simulink model "Hardmon"  (R2025b)
settings: Solver=ode8  StartTime=0.0  StopTime=10  FixedStep=0.0001  RelTol=1e-3
undefined symbols (not defined in the file or in its folder): BMS_Contactor_Command
settings Model: DataDictionary=rev3_data.sldd  Creator=heyka  LastModifiedBy=ryanz
settings DataIOCC: ExternalInput=test_temp.getElement('Temp 1'),test_temp.getElement('Temp 2')  LoadExternalInput=on
settings OptimizationCC: DefaultParameterBehavior=Inlined  EnhancedBackFolding=on  PassReuseOutputArgsThreshold=0.0  ZeroExternalMemoryAtStartup=off  ZeroInternalMemoryAtStartup=off  OptimizeBlockOrder=speed  DifferentSizesBufferReuse=on  OptimizationCustomize=off
settings DebuggingCC: SolverPrmCheckMsg=warning  ParameterTunabilityLossMsg=error  StateNameClashWarn=warning
settings HardwareCC: ProdBitPerInt=16.0  ProdBitPerPointer=16.0  ProdBitPerSizeT=16.0  ProdBitPerPtrDiffT=16.0  ProdLargestAtomicFloat=None  ProdWordSize=16.0  ProdHWDeviceType=STMicroelectronics->ST10/Super10
settings SFSimCC: MATLABDynamicMemAlloc=off  SimTargetLang=C++  SimDLTargetLibrary=mkl-dnn
settings RTWCC: GenCodeOnly=on  Toolchain=MinGW64 | gmake (64-bit Windows)  BuildConfiguration=Faster Runs  TargetLang=C++  GPUComputeCapability=3.5
settings CodeAppCC: ForceParamTrailComments=on  OperatorAnnotations=on  StateflowObjectComments=on
settings GRTTargetCC: TargetLangStandard=C++11 (ISO)  CodeInterfacePackaging=C++ class  SubcomponentCodeInterfacePackaging=C++ class

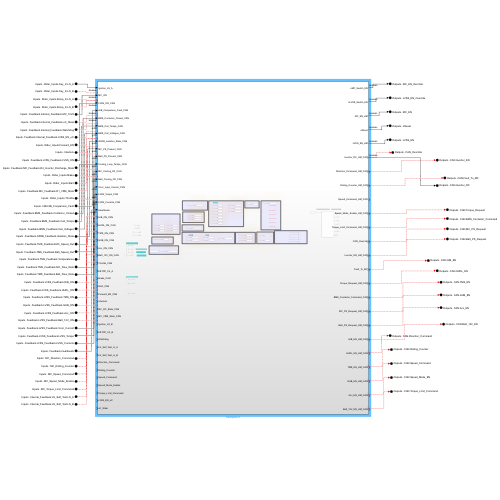
[thumbnail: Simulink's stored preview of the top-level diagram]
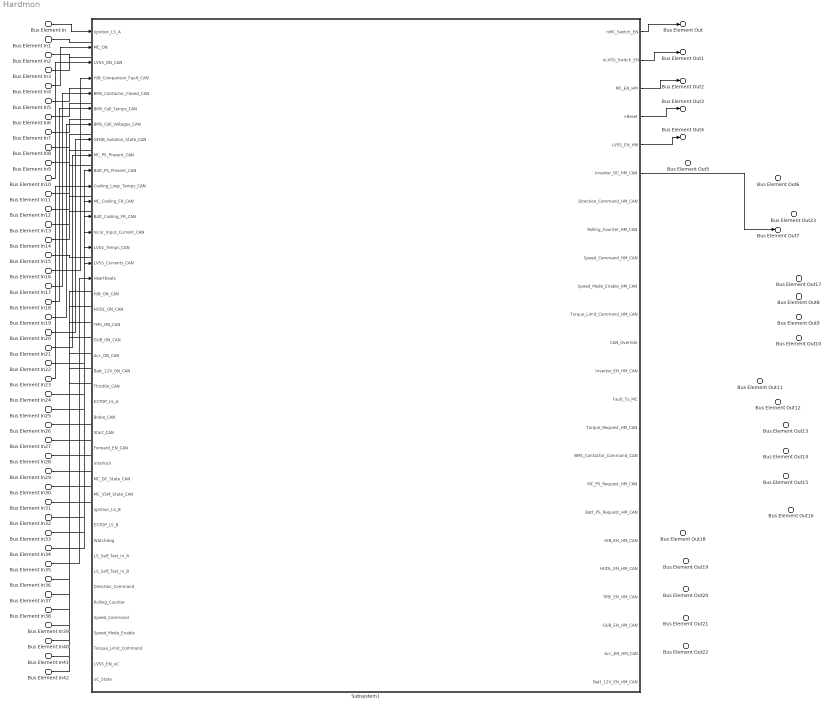
== system Hardmon ==
  Bus Element In2 : Inport  PortName=Inputs  Element=Rider_Inputs.Estop_In.LS_A
  Bus Element In3 : Inport  PortName=Inputs  Element=Rider_Inputs.Estop_In.LS_B
  Bus Element In1 : Inport  PortName=Inputs  Element=Rider_Inputs.Key_In.LS_B
  Bus Element In : Inport  PortName=Inputs  Element=Rider_Inputs.Key_In.LS_A
  Bus Element In8 : Inport  PortName=Inputs  Element=Rider_Inputs.Forward_EN
  Bus Element In12 : Inport  PortName=Inputs  Element=Rider_Inputs.Brake
  Bus Element In13 : Inport  PortName=Inputs  Element=Rider_Inputs.Start
  Bus Element In15 : Inport  PortName=Inputs  Element=Rider_Inputs.Throttle
  Bus Element In4 : Inport  PortName=Inputs  Element=Feedback.Internal_Feedback.MC_12V0
  Bus Element In5 : Inport  PortName=Inputs  Element=Feedback.Internal_Feedback.uC_State
  Bus Element In6 : Inport  PortName=Inputs  Element=Feedback.Internal_Feedback.Watchdog
  Bus Element In7 : Inport  PortName=Inputs  Element=Feedback.Internal_Feedback.LVSS_EN_uC
  Bus Element In10 : Inport  PortName=Inputs  Element=Feedback.LVSS_Feedback.LVSS_ON
  Bus Element In26 : Inport  PortName=Inputs  Element=Feedback.LVSS_Feedback.HIB_ON
  Bus Element In27 : Inport  PortName=Inputs  Element=Feedback.LVSS_Feedback.HUDL_ON
  Bus Element In28 : Inport  PortName=Inputs  Element=Feedback.LVSS_Feedback.TMS_ON
  Bus Element In29 : Inport  PortName=Inputs  Element=Feedback.LVSS_Feedback.GUB_ON
  Bus Element In30 : Inport  PortName=Inputs  Element=Feedback.LVSS_Feedback.Acc_ON
  Bus Element In31 : Inport  PortName=Inputs  Element=Feedback.LVSS_Feedback.Batt_12V_ON
  Bus Element In32 : Inport  PortName=Inputs  Element=Feedback.LVSS_Feedback.Vicor_Current
  Bus Element In33 : Inport  PortName=Inputs  Element=Feedback.LVSS_Feedback.LVSS_Temps
  Bus Element In34 : Inport  PortName=Inputs  Element=Feedback.LVSS_Feedback.LVSS_Currents
  Bus Element In11 : Inport  PortName=Inputs  Element=Feedback.MC_Feedback.D4_Inverter_Discharge_State
  Bus Element In14 : Inport  PortName=Inputs  Element=Feedback.MC_Feedback.D1_VSM_State
  Bus Element In17 : Inport  PortName=Inputs  Element=Feedback.BMS_Feedback.Contactor_Closed
  Bus Element In18 : Inport  PortName=Inputs  Element=Feedback.BMS_Feedback.Cell_Temps
  Bus Element In19 : Inport  PortName=Inputs  Element=Feedback.BMS_Feedback.Cell_Voltages
  Bus Element In20 : Inport  PortName=Inputs  Element=Feedback.GFDB_Feedback.Isolation_State
  Bus Element In21 : Inport  PortName=Inputs  Element=Feedback.TMS_Feedback.MC_Speed_Out
  Bus Element In22 : Inport  PortName=Inputs  Element=Feedback.TMS_Feedback.Batt_Speed_Out
  Bus Element In23 : Inport  PortName=Inputs  Element=Feedback.TMS_Feedback.Temperatures
  Bus Element In24 : Inport  PortName=Inputs  Element=Feedback.TMS_Feedback.MC_Flow_Rate
  Bus Element In25 : Inport  PortName=Inputs  Element=Feedback.TMS_Feedback.Batt_Flow_Rate
  Bus Element In35 : Inport  PortName=Inputs  Element=Feedback.Heartbeats
  Bus Element In9 : Inport  PortName=Inputs  Element=Interlock
  Bus Element In16 : Inport  PortName=Inputs  Element=HIB.HIB_Comparison_Fault
  Bus Element In36 : Inport  PortName=Inputs  Element=MC_Direction_Command
  Bus Element In37 : Inport  PortName=Inputs  Element=MC_Rolling_Counter
  Bus Element In38 : Inport  PortName=Inputs  Element=MC_Speed_Command
  Bus Element In39 : Inport  PortName=Inputs  Element=MC_Speed_Mode_Enable
  Bus Element In40 : Inport  PortName=Inputs  Element=MC_Torque_Limit_Command
  Bus Element In41 : Inport  PortName=Inputs  Element=Internal_Feedback.LS_Self_Test.LS_A
  Bus Element In42 : Inport  PortName=Inputs  Element=Internal_Feedback.LS_Self_Test.LS_B
  Subsystem1 : Subsystem
  Bus Element Out : Outport  PortName=Outputs  Element=MC_EN_Override
  Bus Element Out1 : Outport  PortName=Outputs  Element=LVSS_EN_Override
  Bus Element Out2 : Outport  PortName=Outputs  Element=MC_EN
  Bus Element Out3 : Outport  PortName=Outputs  Element=nReset
  Bus Element Out4 : Outport  PortName=Outputs  Element=LVSS_EN
  Bus Element Out5 : Outport  PortName=Outputs  Element=CAN_Override
  Bus Element Out6 : Outport  PortName=Outputs  Element=CAN.Inverter_EN
  Bus Element Out23 : Outport  PortName=Outputs  Element=CAN.Fault_To_MC
  Bus Element Out7 : Outport  PortName=Outputs  Element=CAN.Inverter_DC
  Bus Element Out17 : Outport  PortName=Outputs  Element=CAN.Torque_Request
  Bus Element Out8 : Outport  PortName=Outputs  Element=CAN.BMS_Contactor_Command
  Bus Element Out9 : Outport  PortName=Outputs  Element=CAN.MC_PS_Request
  Bus Element Out10 : Outport  PortName=Outputs  Element=CAN.Batt_PS_Request
  Bus Element Out11 : Outport  PortName=Outputs  Element=CAN.HIB_EN
  Bus Element Out12 : Outport  PortName=Outputs  Element=CAN.HUDL_EN
  Bus Element Out13 : Outport  PortName=Outputs  Element=CAN.TMS_EN
  Bus Element Out14 : Outport  PortName=Outputs  Element=CAN.GUB_EN
  Bus Element Out15 : Outport  PortName=Outputs  Element=CAN.Acc_EN
  Bus Element Out16 : Outport  PortName=Outputs  Element=CAN.Batt_12V_EN
  Bus Element Out18 : Outport  PortName=Outputs  Element=CAN.Direction_Command
  Bus Element Out19 : Outport  PortName=Outputs  Element=CAN.Rolling_Counter
  Bus Element Out20 : Outport  PortName=Outputs  Element=CAN.Speed_Command
  Bus Element Out21 : Outport  PortName=Outputs  Element=CAN.Speed_Mode_EN
  Bus Element Out22 : Outport  PortName=Outputs  Element=CAN.Torque_Limit_Command
  wires:
  Bus Element In/1 -> Subsystem1/1(Ignition_LS_A)
  Bus Element In1/1 -> ?
  Bus Element In2/1 -> ?
  Bus Element In3/1 -> ?
  Bus Element In4/1 -> Subsystem1/2(MC_ON)
  Bus Element In5/1 -> ?
  Bus Element In6/1 -> ?
  Bus Element In7/1 -> ?
  Bus Element In8/1 -> ?
  Bus Element In9/1 -> ?
  Bus Element In10/1 -> Subsystem1/3(LVSS_ON_CAN)
  Bus Element In11/1 -> ?
  Bus Element In12/1 -> ?
  Bus Element In13/1 -> ?
  Bus Element In14/1 -> ?
  Bus Element In15/1 -> ?
  Bus Element In16/1 -> Subsystem1/4(HIB_Comparison_Fault_CAN)
  Bus Element In17/1 -> Subsystem1/5(BMS_Contactor_Closed_CAN)
  Bus Element In18/1 -> Subsystem1/6(BMS_Cell_Temps_CAN)
  Bus Element In19/1 -> Subsystem1/7(BMS_Cell_Voltages_CAN)
  Bus Element In20/1 -> Subsystem1/8(GFDB_Isolation_State_CAN)
  Bus Element In21/1 -> Subsystem1/9(MC_PS_Present_CAN)
  Bus Element In22/1 -> Subsystem1/10(Batt_PS_Present_CAN)
  Bus Element In23/1 -> Subsystem1/11(Cooling_Loop_Temps_CAN)
  Bus Element In24/1 -> Subsystem1/12(MC_Cooling_FR_CAN)
  Bus Element In25/1 -> Subsystem1/13(Batt_Cooling_FR_CAN)
  Bus Element In26/1 -> ?
  Bus Element In27/1 -> ?
  Bus Element In28/1 -> ?
  Bus Element In29/1 -> ?
  Bus Element In30/1 -> ?
  Bus Element In31/1 -> ?
  Bus Element In32/1 -> Subsystem1/14(Vicor_Input_Current_CAN)
  Bus Element In33/1 -> Subsystem1/15(LVSS_Temps_CAN)
  Bus Element In34/1 -> Subsystem1/16(LVSS_Currents_CAN)
  Bus Element In35/1 -> Subsystem1/17(Heartbeats)
  Bus Element In36/1 -> ?
  Bus Element In37/1 -> ?
  Bus Element In38/1 -> ?
  Bus Element In39/1 -> ?
  Bus Element In40/1 -> ?
  Bus Element In41/1 -> ?
  Bus Element In42/1 -> ?
  Subsystem1/1(nMC_Switch_EN) -> Bus Element Out/1
  Subsystem1/2(nLVSS_Switch_EN) -> Bus Element Out1/1
  Subsystem1/3(MC_EN_HM) -> Bus Element Out2/1
  Subsystem1/4(nReset) -> Bus Element Out3/1
  Subsystem1/5(LVSS_EN_HM) -> Bus Element Out4/1
  ? -> Bus Element Out5/1
  ? -> Bus Element Out6/1
  Subsystem1/6(Inverter_DC_HM_CAN) -> Bus Element Out7/1
  ? -> Bus Element Out8/1
  ? -> Bus Element Out9/1
  ? -> Bus Element Out10/1
  ? -> Bus Element Out11/1
  ? -> Bus Element Out12/1
  ? -> Bus Element Out13/1
  ? -> Bus Element Out14/1
  ? -> Bus Element Out15/1
  ? -> Bus Element Out16/1
  ? -> Bus Element Out17/1
  ? -> Bus Element Out18/1
  ? -> Bus Element Out19/1
  ? -> Bus Element Out20/1
  ? -> Bus Element Out21/1
  ? -> Bus Element Out22/1
  ? -> Bus Element Out23/1

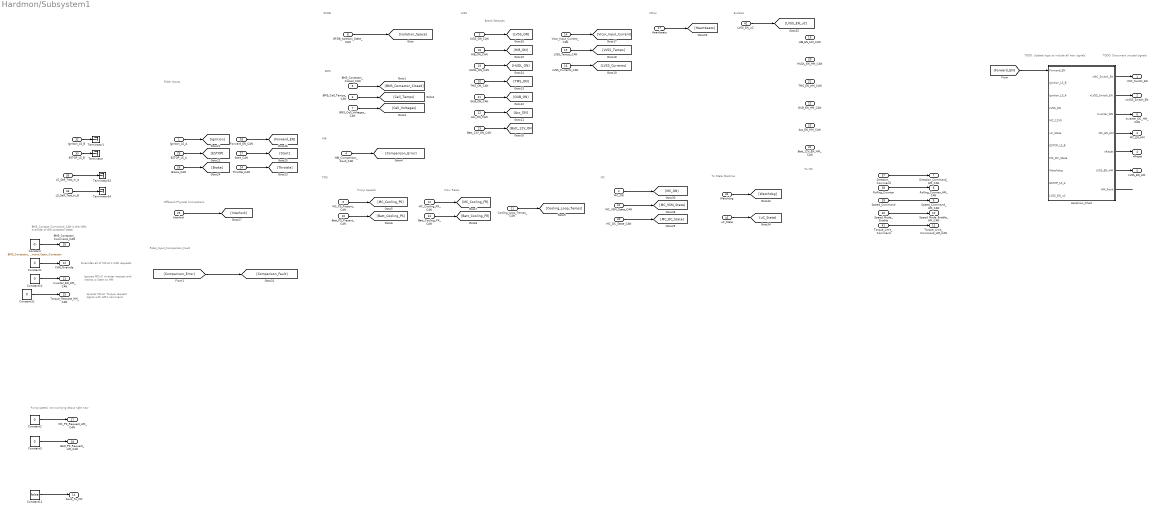
== system Hardmon/Subsystem1 ==
  note: Ignores MCuC inverter request and makes is listen to HM
  note: Overrides all of MCuC's CAN requests
  note: Pump speed, not worrying about right now
  note: BMS_Contact_Command_CAN
      | is the HMs override of the contactor state.
  note: Rider_Input_Comparison_Fault
  note: To MC
  note: To State Machine
  note: MC
  note: Offboard Physical Connections
  note: Rider Inputs
  note: Enables
  note: Other
  note: Board Statuses
  note: LVSS
  note: Pump Speeds
  note: TMS
  note: HIB
  note: BMS
  note: GFDB
  note: TODO: Update logic to include all new signals
  note: TODO: Document unused signals
  note: Flow Rates
  note: Ignores MCuC Torque request signal with HM's command
  Ignition_LS_A : Inport  OutDataTypeStr=boolean
  MC_ON : Inport  Port=2  OutDataTypeStr=boolean
  LVSS_ON_CAN : Inport  Port=3  OutDataTypeStr=boolean
  HIB_Comparison_Fault_CAN : Inport  Port=4  OutDataTypeStr=boolean
  BMS_Contactor_Closed_CAN : Inport  Port=5  OutDataTypeStr=boolean
  BMS_Cell_Temps_CAN : Inport  Port=6  OutDataTypeStr=int32  PortDimensions=[1,45]
  BMS_Cell_Voltages_CAN : Inport  Port=7  OutDataTypeStr=int16  PortDimensions=[1,100]
  GFDB_Isolation_State_CAN : Inport  Port=8  OutDataTypeStr=uint8
  MC_PS_Present_CAN : Inport  Port=9  OutDataTypeStr=uint8
  Batt_PS_Present_CAN : Inport  Port=10  OutDataTypeStr=uint8
  Cooling_Loop_Temps_CAN : Inport  Port=11  OutDataTypeStr=int32  PortDimensions=[1,5]
  MC_Cooling_FR_CAN : Inport  Port=12  OutDataTypeStr=int16
  Batt_Cooling_FR_CAN : Inport  Port=13  OutDataTypeStr=int16
  Vicor_Input_Current_CAN : Inport  Port=14  OutDataTypeStr=int16
  LVSS_Temps_CAN : Inport  Port=15  OutDataTypeStr=int32  PortDimensions=[1,6]
  LVSS_Currents_CAN : Inport  Port=16  OutDataTypeStr=int16  PortDimensions=[1,6]
  Heartbeats : Inport  Port=17  OutDataTypeStr=uint32  PortDimensions=[1,5]
  HIB_ON_CAN : Inport  Port=18  OutDataTypeStr=boolean
  HUDL_ON_CAN : Inport  Port=19  OutDataTypeStr=boolean
  TMS_ON_CAN : Inport  Port=20  OutDataTypeStr=boolean
  GUB_ON_CAN : Inport  Port=21  OutDataTypeStr=boolean
  Acc_ON_CAN : Inport  Port=22  OutDataTypeStr=boolean
  Batt_12V_ON_CAN : Inport  Port=23  OutDataTypeStr=boolean
  Throttle_CAN : Inport  Port=24  OutDataTypeStr=int16
  ESTOP_LS_A : Inport  Port=25  OutDataTypeStr=boolean
  Brake_CAN : Inport  Port=26  OutDataTypeStr=boolean
  Start_CAN : Inport  Port=27  OutDataTypeStr=boolean
  Forward_EN_CAN : Inport  Port=28  OutDataTypeStr=boolean
  Interlock : Inport  Port=29  OutDataTypeStr=boolean
  MC_DC_State_CAN : Inport  Port=30  OutDataTypeStr=Enum: MC_DC_State
  MC_VSM_State_CAN : Inport  Port=31  OutDataTypeStr=Enum: MC_VSM_State
  Ignition_LS_B : Inport  Port=32  OutDataTypeStr=boolean
  ESTOP_LS_B : Inport  Port=33  OutDataTypeStr=boolean
  Watchdog : Inport  Port=34  OutDataTypeStr=boolean
  LS_Self_Test_In_A : Inport  Port=35  OutDataTypeStr=boolean
  LS_Self_Test_In_B : Inport  Port=36  OutDataTypeStr=boolean
  Direction_Command : Inport  Port=37  OutDataTypeStr=int16
  Rolling_Counter : Inport  Port=38  OutDataTypeStr=int16
  Speed_Command : Inport  Port=39  OutDataTypeStr=int16
  Speed_Mode_Enable : Inport  Port=40  OutDataTypeStr=int16
  Torque_Limit_Command : Inport  Port=41  OutDataTypeStr=int16
  LVSS_EN_uC : Inport  Port=42  OutDataTypeStr=boolean
  uC_State : Inport  Port=43  OutDataTypeStr=Enum: UC_State
  Constant : Constant  Value=BMS_Contactor_Command.Open_Contactor  OutDataTypeStr=Enum: BMS_Contactor_Command
  Constant1 : Constant  Value=0  OutDataTypeStr=boolean
  Constant10 : Constant  Value=0  OutDataTypeStr=boolean
  Constant11 : Constant  Value=0  OutDataTypeStr=int16
  Constant12 : Constant  Value=false  OutDataTypeStr=boolean
  Constant2 : Constant  Value=0  OutDataTypeStr=uint8
  Constant3 : Constant  Value=0  OutDataTypeStr=uint8
  Hardmon_Chart : Stateflow chart  TreatAsAtomicUnit=on
      settings: PortSchema="{\"entries\":[{\"content\":{\"sides\":[{\"content\":{\"connectorIds\":[\"In1\",\"In2\",\"In3\",\"In4\",\"In5\",\"In6\",\"In7\",\"In8\",\"In9\",\"In10\",\"In11\"]},\"type\":\"ConnectorPlacement.EquallySpacedRectSide\",\"uuid\":\"6d1a41ef-67e8-41d6-9adb-1761831f6d0e\"},{\"content\":{\"connectorIds\":[\"Out1\",\"Out7\",\"Out2\",\"Out3\",\"Out4\",\"Out5\",\"Out6\"],\"side\":\"RIGHT\"},\"type\":\"ConnectorPlacement.EquallySpacedRectSide\",\"uuid\":\"1c1f5b1f-9a19-48ee-ac61-8a13c1cfd4a8\"},{\"content\":{\"side\":\"TOP\"},\"type\":\"ConnectorPlacement.EquallySpacedRectSide\",\"uuid\":\"7f8ec887-50f7-4fb3-9eed-5aef04cf2afb\"}]},\"type\":\"ConnectorPlacement.EquallySpacedConnector\",\"uuid\":\"822c8876-1e52-4482-83f3-7114ae95ed93\"}],\"packageUris\":[\"http://schema.mathworks.com/mf0/Connector/R2020b\"],\"version\":\"1.0\"}"
  Terminator{,1,33..34} (4 alike) : Terminator
  nMC_Switch_EN : Outport  OutDataTypeStr=boolean
  nLVSS_Switch_EN : Outport  Port=2  OutDataTypeStr=boolean
  MC_EN_HM : Outport  Port=3  OutDataTypeStr=boolean
  nReset : Outport  Port=4  OutDataTypeStr=boolean
  LVSS_EN_HM : Outport  Port=5  OutDataTypeStr=boolean
  Inverter_DC_HM_CAN : Outport  Port=6  OutDataTypeStr=boolean
  Direction_Command_HM_CAN : Outport  Port=7  OutDataTypeStr=int16
  Rolling_Counter_HM_CAN : Outport  Port=8  OutDataTypeStr=int16
  Speed_Command_HM_CAN : Outport  Port=9  OutDataTypeStr=int16
  Speed_Mode_Enable_HM_CAN : Outport  Port=10  OutDataTypeStr=int16
  Torque_Limit_Command_HM_CAN : Outport  Port=11  OutDataTypeStr=int16
  CAN_Override : Outport  Port=12  OutDataTypeStr=boolean
  Inverter_EN_HM_CAN : Outport  Port=13  OutDataTypeStr=boolean
  Fault_To_MC : Outport  Port=14  OutDataTypeStr=boolean
  Torque_Request_HM_CAN : Outport  Port=15  OutDataTypeStr=int16
  BMS_Contactor_Command_CAN : Outport  Port=16  OutDataTypeStr=Enum: BMS_Contactor_Command
  MC_PS_Request_HM_CAN : Outport  Port=17
  Batt_PS_Request_HM_CAN : Outport  Port=18
  HIB_EN_HM_CAN : Outport  Port=19  OutDataTypeStr=boolean
  HUDL_EN_HM_CAN : Outport  Port=20  OutDataTypeStr=boolean
  TMS_EN_HM_CAN : Outport  Port=21  OutDataTypeStr=boolean
  GUB_EN_HM_CAN : Outport  Port=22  OutDataTypeStr=boolean
  Acc_EN_HM_CAN : Outport  Port=23  OutDataTypeStr=boolean
  Batt_12V_EN_HM_CAN : Outport  Port=24  OutDataTypeStr=boolean
  wires:
  Vicor_Input_Current_CAN/1 -> [Vicor_Input_Current]
  LVSS_Temps_CAN/1 -> [LVSS_Temps]
  MC_PS_Present_CAN/1 -> [MC_Cooling_PS]
  Heartbeats/1 -> [Heartbeats]
  BMS_Cell_Temps_CAN/1 -> [Cell_Temps]
  Hardmon_Chart/1(nMC_Switch_EN) -> nMC_Switch_EN/1
  LVSS_Currents_CAN/1 -> [LVSS_Currents]
  BMS_Cell_Voltages_CAN/1 -> [Cell_Voltages]
  Hardmon_Chart/4(nReset) -> nReset/1
  MC_Cooling_FR_CAN/1 -> [MC_Cooling_FR]
  Batt_PS_Present_CAN/1 -> [Batt_Cooling_PS]
  Batt_Cooling_FR_CAN/1 -> [Batt_Cooling_FR]
  HIB_Comparison_Fault_CAN/1 -> [Comparison_Error]
  BMS_Contactor_Closed_CAN/1 -> [BMS_Contactor_Closed]
  Hardmon_Chart/7(nLVSS_Switch_EN) -> nLVSS_Switch_EN/1
  Hardmon_Chart/2(Inverter_DIS) -> Inverter_DC_HM_CAN/1
  Cooling_Loop_Temps_CAN/1 -> [Cooling_Loop_Temps]
  GFDB_Isolation_State_CAN/1 -> [Isolation_Space]
  Hardmon_Chart/5(LVSS_EN_HM) -> LVSS_EN_HM/1
  Hardmon_Chart/3(MC_EN_HM) -> MC_EN_HM/1
  Hardmon_Chart/6(HM_Fault) -> ?
  TMS_ON_CAN/1 -> [TMS_ON]
  Acc_ON_CAN/1 -> [Acc_ON]
  Batt_12V_ON_CAN/1 -> [Batt_12V_ON]
  HUDL_ON_CAN/1 -> [HUDL_ON]
  HIB_ON_CAN/1 -> [HIB_ON]
  GUB_ON_CAN/1 -> [GUB_ON]
  LVSS_ON_CAN/1 -> [LVSS_ON]
  Ignition_LS_A/1 -> [Ignition]
  ESTOP_LS_A/1 -> [ESTOP]
  Throttle_CAN/1 -> [Throttle]
  Brake_CAN/1 -> [Brake]
  Start_CAN/1 -> [Start]
  Forward_EN_CAN/1 -> [Forward_EN]
  Interlock/1 -> [Interlock]
  MC_DC_State_CAN/1 -> [MC_DC_State]
  MC_VSM_State_CAN/1 -> [MC_VSM_State]
  MC_ON/1 -> [MC_ON]
  [Forward_EN] -> Hardmon_Chart/1(Forward_EN)
  LS_Self_Test_In_B/1 -> Terminator34/1
  LS_Self_Test_In_A/1 -> Terminator33/1
  Speed_Command/1 -> Speed_Command_HM_CAN/1
  Torque_Limit_Command/1 -> Torque_Limit_Command_HM_CAN/1
  Rolling_Counter/1 -> Rolling_Counter_HM_CAN/1
  Direction_Command/1 -> Direction_Command_HM_CAN/1
  Speed_Mode_Enable/1 -> Speed_Mode_Enable_HM_CAN/1
  Watchdog/1 -> [Watchdog]
  Constant10/1 -> Inverter_EN_HM_CAN/1
  Constant12/1 -> Fault_To_MC/1
  Constant/1 -> BMS_Contactor_Command_CAN/1
  Constant3/1 -> Batt_PS_Request_HM_CAN/1
  Constant1/1 -> CAN_Override/1
  Constant2/1 -> MC_PS_Request_HM_CAN/1
  Constant11/1 -> Torque_Request_HM_CAN/1
  [Comparison_Error] -> [Comparison_Fault]
  LVSS_EN_uC/1 -> [LVSS_EN_uC]
  ? -> HIB_EN_HM_CAN/1
  ? -> TMS_EN_HM_CAN/1
  ? -> Batt_12V_EN_HM_CAN/1
  ? -> GUB_EN_HM_CAN/1
  ? -> HUDL_EN_HM_CAN/1
  ? -> Acc_EN_HM_CAN/1
  uC_State/1 -> [uC_State]
  Ignition_LS_B/1 -> Terminator1/1
  ESTOP_LS_B/1 -> Terminator/1

== stateflow chart Hardmon/Subsystem1/Hardmon_Chart ==
  note: Need to update State machine to show the proper HM signals
  state Logic
    state LVSS_MC_Startup
      entry:
      MC_Uncharged = false;
      uC_State = UC_State.LVSS_MC_Startup;
      LVSS_EN_uC = true;
      MC_EN = true;
    state MC_Off
      entry:
      MC_EN = false;
      LVSS_EN_uC = false;
      uC_State = UC_State.MC_Off;
      MC_Uncharged = true;
      Inverter_EN = false;
    state LVSS_MC_Shutdown
      entry:
      uC_State = UC_State.LVSS_MC_Shutdown;
      LVSS_EN_uC = false;
      MC_EN = false;
    state Preset
      entry:
      uC_State = UC_State.Preset;
      Batt_Contactor = BMS_Contactor_Command.Open_Contactor;
      exit:
      Self_Test = false;
      MC_Self_Test = false
      state MC_ST
        entry:
        Self_Test = true;
        MC_Self_Test = true;
        state MC_EN_ON
          entry:
          MC_EN = true;
        state MC_EN_OFF
          entry:
          MC_EN = false;
        (default) -> MC_EN_ON
        MC_EN_ON -> MC_EN_OFF : [MC_ON == true]
      (default) -> MC_ST
    state MC_Init
      entry:
      uC_State = UC_State.MC_Init;
      Batt_12V_EN = true;
      TMS_EN = true;
      HIB_EN = true;
      HUDL_EN = true;
      GUB_EN = true;
      Acc_EN = true;
    state MC_Discharging
      entry:
      uC_State = UC_State.MC_Discharging;
      exit:
      MC_Uncharged = true;
      Inverter_DC = false;
    state ESTOP
      entry:
      uC_State = UC_State.Estop;
      Batt_Contactor = BMS_Contactor_Command.Open_Contactor;
      LVSS_EN_uC = false;
      Activate_ESTOP = false;
    state Key_Cycle
      entry:
      uC_State = UC_State.Key_Cycle;
      Batt_Contactor = BMS_Contactor_Command.Close_Contactor;
    state Contactor_Closed
      entry:
      uC_State = UC_State.Contactor_Closed;
      Inverter_EN = false;
    state Contactor_Open
      entry:
      Inverter_EN = false;
      Inverter_DC = true;
      uC_State = UC_State.Contactor_Open;
      Acc_EN = false;
      GUB_EN = false;
      HUDL_EN = false;
      HIB_EN = false;
      TMS_EN = false;
      Batt_12V_EN = false;
    state Fault
      entry:
      uC_State = UC_State.Fault;
      Activate_Fault = false;
      Fault = true;
      Batt_Contactor = BMS_Contactor_Command.Stay;
      exit:
      Fault = false;
    state Super_Fault
      entry:
      uC_State = UC_State.Super_Fault;
      Batt_Contactor = BMS_Contactor_Command.Open_Contactor;
      Super_Super_Fault = true;
    state MC_Ready
      entry:
      uC_State = UC_State.MC_Ready;
      Inverter_EN = false;
    state MC_Active
      entry:
      Inverter_EN = true;
      uC_State = UC_State.MC_Active;
      Torque_Request = 0;
      during:
      Torque_Request = Throttle;
      end
      exit:
      Torque_Request = 0;
    LVSS_MC_Shutdown -> MC_Off : [MC_ON == false && LVSS_ON == false]
    (default) -> Preset
    MC_Off -> LVSS_MC_Startup : [Ignition == true]
    LVSS_MC_Startup -> MC_Init : [MC_ON == true && LVSS_ON == true]
    MC_Discharging -> LVSS_MC_Shutdown : [MC_Current_DC_State == MC_DC_State.Complete]
    Key_Cycle -> MC_Off : [Ignition == false]
    Preset -> Key_Cycle : [Leave_Preset == true]
    MC_Init -> Contactor_Open [order 1] : [Ignition == false]
    ESTOP -> Key_Cycle : [ESTOP == false]
    Logic -> ESTOP [order 3] : [ESTOP == true && MC_Uncharged == true && uC_State ~= UC_State.Preset]
    Contactor_Open -> MC_Discharging : [MC_Current_DC_State ~= MC_DC_State.Disabled]
    MC_Init -> Contactor_Closed [order 2] : [MC_Current_VSM_State == MC_VSM_State.Ready]
    Fault -> Key_Cycle : [STO == true]
    Logic -> Contactor_Open [order 2] : [Super_Fault == true && MC_Uncharged == false && Activate_Super_Fault == false]{Activate_Super_Fault = true;}
    Contactor_Closed -> Contactor_Open [order 1] : [Ignition == false]
    Logic -> Contactor_Open [order 4] : [ESTOP == true && MC_Uncharged == false && Activate_ESTOP == false]{Activate_ESTOP = true;}
    Logic -> Fault [order 5] : [STO == false && MC_Uncharged == true]
    Logic -> Contactor_Open [order 6] : [STO == false && MC_Uncharged == false && Activate_Fault == false]{Activate_Fault = true;}
    Contactor_Closed -> MC_Ready [order 2] : [Start == true]
    MC_Active -> Contactor_Open [order 2] : [Ignition == false]
    MC_Ready -> MC_Active : [Activate_MC == true]
    Logic -> Super_Fault [order 1] : [(Super_Fault == true && MC_Uncharged == true) || Super_Super_Fault == true]
    MC_Active -> MC_Ready [order 1] : [Forward_EN == false]
  data: WD_Counter local; Forward_EN input; Ignition_LS_B input; Ignition_LS_A input; LVSS_ON input; MC_12V0 input; uC_State input; nMC_Switch_EN output; Inverter_DIS output; MC_EN_HM output; nReset output =true; ESTOP_State_Counter local; Ignition_State_Counter local; Invalid_State_Counter local; LVSS_Counter local; LVSS_EN_HM output; ESTOP_LS_B input; MC_DC_State input; Watchdog input; ESTOP_Counter local; ESTOP_LS_A input =0; HM_Fault output; LVSS_EN_uC input; nLVSS_Switch_EN output
